simulink model "A421_FP_pt2_model"  (R2022b)
settings: Solver=VariableStepAuto  StartTime=0.0  StopTime=6000  RelTol=1e-3
values from neighbouring files (symbols this model uses):
  initialState = [W_b_ECI;princpRot_b_ECI;epsilon_b_ECI;eta_b_ECI]    [A421_torqueFreeMotion.m]
  Torque = 0    [A421_torqueFreeMotion.m]
undefined symbols (not defined in the file or in its folder): InertiaMatrix
settings Model: Creator=willb  LastModifiedBy=willb

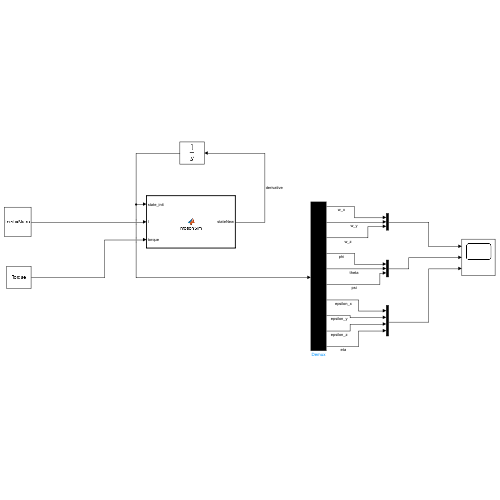
[thumbnail: Simulink's stored preview of the top-level diagram]
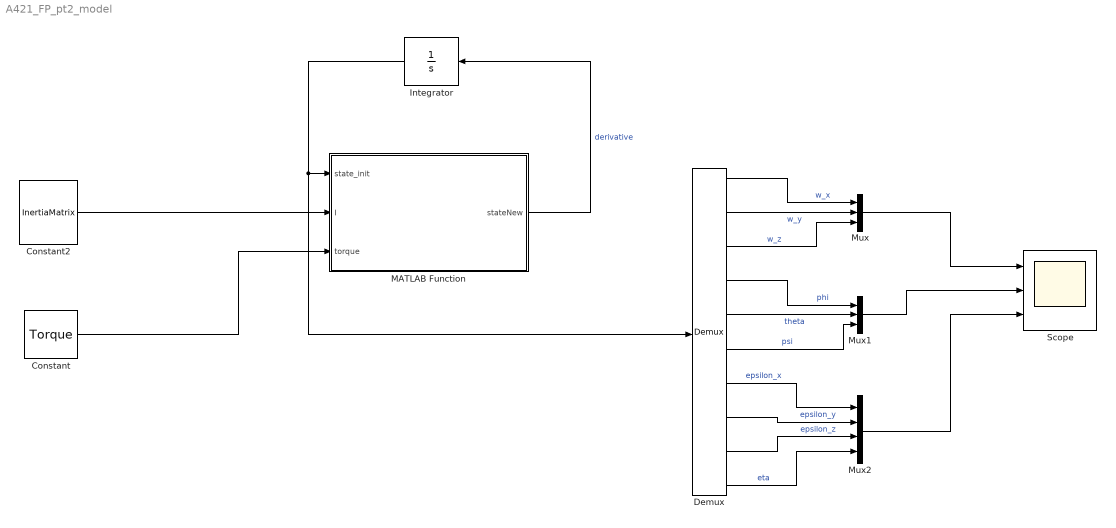
== system A421_FP_pt2_model ==
  Constant : Constant  Value=Torque
  Constant2 : Constant  Value=InertiaMatrix
  Demux : Demux  Outputs=10
  Integrator : Integrator  InitialCondition=initialState
  MATLAB Function : MATLAB Function  TreatAsAtomicUnit=on
  Mux : Mux  Inputs=3
  Mux1 : Mux  Inputs=3
  Mux2 : Mux
  Scope : Scope  NumInputPorts=3
  wires:
  Constant/1 -> MATLAB Function/3(torque)
  Constant2/1 -> MATLAB Function/2(I)
  MATLAB Function/1(stateNew) -> Integrator/1  "derivative"
  Integrator/1 -> Demux/1, MATLAB Function/1(state_init)
  Demux/1 -> Mux/1  "w_x"
  Demux/2 -> Mux/2  "w_y"
  Demux/3 -> Mux/3  "w_z"
  Demux/4 -> Mux1/1  "phi"
  Demux/5 -> Mux1/2  "theta"
  Demux/6 -> Mux1/3  "psi"
  Demux/7 -> Mux2/1  "epsilon_x"
  Demux/8 -> Mux2/2  "epsilon_y"
  Demux/9 -> Mux2/3  "epsilon_z"
  Demux/10 -> Mux2/4  "eta"
  Mux/1 -> Scope/1
  Mux1/1 -> Scope/2
  Mux2/1 -> Scope/3

== matlab function A421_FP_pt2_model/MATLAB Function ==
  data: stateNew output; state_init input; I input; torque input
function stateNew  = motionSim(state_init,I,torque)
% Inputs
    % time
    % state init = [wx,wy,wz,phi,theta,psi,epsilonx,epsilony,epsilonz,eta]
    % I = inertia matrix
    % torque
% Ouput
    % stateNew = derivative of stateInit
% *All angles in RADIANS*

% Angular Velocity
w_init = state_init(1:3);    
wx = w_init(1);
wy = w_init(2);
wz = w_init(3);
wcross = [0, -wz, wy; wz, 0, -wx; -wy, wx, 0];

w_dot = (I^-1)*(-wcross*I*w_init+torque);

% Euler Angles
initEuler = state_init(4:6);
phi = initEuler(1);
theta = initEuler(2);
psi = initEuler(3);

[Euler_dot] = (1/cos(theta))*...
    [cos(theta), sin(phi)*sin(theta), cos(phi)*sin(theta);...
     0,          cos(phi)*cos(theta), -sin(phi)*cos(theta);...
     0,          sin(phi), cos(phi)]*w_init;

% Quaternion
epsilon0 = state_init(7:9);
eta0 = state_init(10);
epsilCross = [          0, -epsilon0(3),  epsilon0(2); ...
              epsilon0(3),            0, -epsilon0(1); ...
             -epsilon0(2),  epsilon0(1),            0];

epsilonDot = 0.5*(eta0*eye(3) + epsilCross)*w_init;
etaDot = -0.5*epsilon0'*w_init;

stateNew = [w_dot;Euler_dot;epsilonDot;etaDot];
end
